simulink model "benchmark_2"  (R2016a)
settings: Solver=VariableStepAuto  StartTime=0.0  StopTime=time  RelTol=1e-3
values from neighbouring files (symbols this model uses):
  time_step = 0.01    [UAV_LAUNCHER_ASY_working_prot__v10.m]    (also in matlab_calc_actuator.m = 0.1; matlab_calc_tank_side.m = 7.0175)
libraries: fl_lib x10, nesl_utility x4
settings Model: Creator=Engr.Hammad  LastModifiedBy=Engr.Hammad

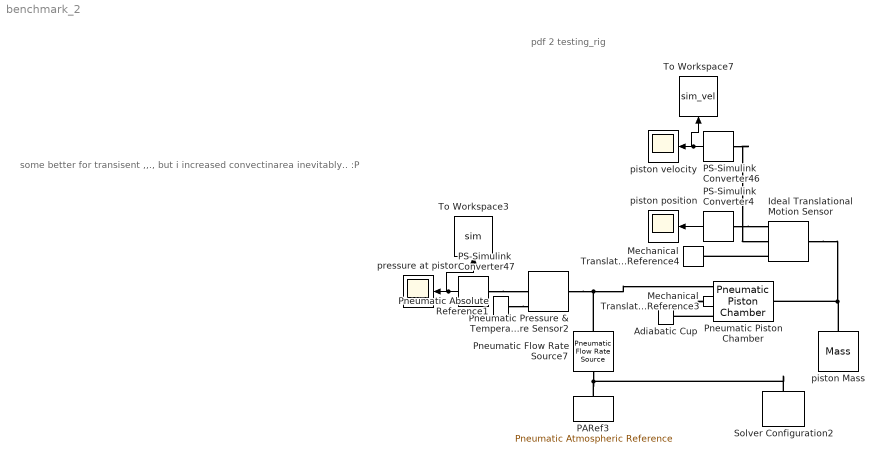
== system benchmark_2 ==
  note: some better for transisent ,,., but i increased convectinarea inevitably.. :P
  note: pdf 2 testing_rig
  Adiabatic Cup : fl_lib/Pneumatic/Pneumatic Elements/Adiabatic Cup
  Ideal Translational Motion Sensor : fl_lib/Mechanical/Mechanical Sensors/Ideal Translational Motion Sensor  offset=0 m
  Mechanical Translational Reference3 : fl_lib/Mechanical/Translational Elements/Mechanical Translational Reference
  Mechanical Translational Reference4 : fl_lib/Mechanical/Translational Elements/Mechanical Translational Reference
  PARef3 : fl_lib/Pneumatic/Pneumatic Elements/Pneumatic Atmospheric Reference
  PS-Simulink Converter4 : nesl_utility/PS-Simulink Converter  PhysicalDomain=network_engine_domain  SubClassName=ps_output  LeftPortType=input  RightPortType=output  PseudoPeriodic=off  Frequencies=[]  Unit=1  AffineConversion=off
  PS-Simulink Converter46 : nesl_utility/PS-Simulink Converter  PhysicalDomain=network_engine_domain  SubClassName=ps_output  LeftPortType=input  RightPortType=output  PseudoPeriodic=off  Frequencies=[]  Unit=1  AffineConversion=off
  PS-Simulink Converter47 : nesl_utility/PS-Simulink Converter  PhysicalDomain=network_engine_domain  SubClassName=ps_output  LeftPortType=input  RightPortType=output  PseudoPeriodic=off  Frequencies=[]  Unit=1  AffineConversion=off
  Pneumatic Absolute Reference1 : fl_lib/Pneumatic/Pneumatic Elements/Pneumatic Absolute Reference
  Pneumatic Flow Rate Source7 : fl_lib/Pneumatic/Pneumatic Sources/Pneumatic Flow Rate Source  gas_flow_reference=G kg/s
  Pneumatic Piston Chamber : fl_lib/Pneumatic/Pneumatic Elements/Pneumatic Piston Chamber  Area=pis_area m^2  x0=0 m  V0=1e-5 m^3  or=1  pressure_specify=on  pressure_priority=High  pressure=1.01325e+5 Pa  temperature_specify=off  temperature_priority=High  temperature=300 K  gas_flow_specify=off  gas_flow_priority=None  gas_flow=0 kg/s  heat_flow_specify=off  heat_flow_priority=None  heat_flow=0 J/s  heat_exch_flow_specify=off  heat_exch_flow_priority=None  heat_exch_flow=0 J/s  velocity_specify=off  velocity_priority=None  velocity=0 m/s  force_specify=off  force_priority=None  force=0 N
  Pneumatic Pressure & Temperature Sensor2 : fl_lib/Pneumatic/Pneumatic Sensors/Pneumatic Pressure & Temperature Sensor
  Solver Configuration2 : nesl_utility/Solver Configuration  PhysicalDomain=network_engine_domain  SubClassName=solver  LeftPortType=input  RightPortType=generic  Accelerate=off  Tones=[]  Harmonics=[]  SimulateNoise=off  Profile=off  UseLocalSampling=off  EnableSwitchedLinearOptims=on  FrequencyDomain=off  UseCCode=off  RelTol=0.001  AbsTol=1e-06  MinStep=1e-09  ToWorkspace=off  RevertToSquareIcSolve=off  NumHomotopyIterations=100  PhasorMode=off  PhasorModeNumHarmonics=1  OverrideAbsTol=off  DoDC=off  ResidualTolerance=1e-09  UseLocalSolver=off  LocalSolverChoice=NE_BACKWARD_EULER_ADVANCER  LocalSolverSampleTime=0.001  DoFixedCost=off  MaxNonlinIter=3  MaxModeIter=2  LinearAlgebra=Sparse  DelaysMemoryBudget=1024  AutomaticFiltering=on  FilteringTimeConstant=0.001
  To Workspace3 : ToWorkspace  VariableName=sim  SaveFormat=Structure With Time  SampleTime=time_step
  To Workspace7 : ToWorkspace  VariableName=sim_vel  SaveFormat=Structure With Time  SampleTime=time_step
  piston position : Scope
  piston Mass : fl_lib/Mechanical/Translational Elements/Mass  mass=1 kg  v_specify=off  v_priority=High  v=0 m/s  f_specify=off  f_priority=None  f=0 N
  piston velocity : Scope
  pressure at piston : Scope
  wires:
  PS-Simulink Converter4/1 -> piston position/1
  PS-Simulink Converter46/1 -> To Workspace7/1, piston velocity/1
  PS-Simulink Converter47/1 -> To Workspace3/1, pressure at piston/1
  connections:
  Pneumatic Flow Rate Source7/RConn1 -- PARef3/LConn1 -- Solver Configuration2/RConn1
  piston Mass/LConn1 -- Pneumatic Piston Chamber/RConn1 -- Ideal Translational Motion Sensor/LConn1
  Pneumatic Pressure & Temperature Sensor2/LConn1 -- Pneumatic Piston Chamber/LConn1 -- Pneumatic Flow Rate Source7/LConn1
  Pneumatic Piston Chamber/LConn3 -- Adiabatic Cup/LConn1
  PS-Simulink Converter47/LConn1 -- Pneumatic Pressure & Temperature Sensor2/RConn2
  PS-Simulink Converter46/LConn1 -- Ideal Translational Motion Sensor/RConn2
  Pneumatic Absolute Reference1/LConn1 -- Pneumatic Pressure & Temperature Sensor2/RConn1
  Ideal Translational Motion Sensor/RConn1 -- Mechanical Translational Reference4/LConn1
  PS-Simulink Converter4/LConn1 -- Ideal Translational Motion Sensor/RConn3
  Pneumatic Piston Chamber/LConn2 -- Mechanical Translational Reference3/LConn1
